simulink model "LuGre_model_BAFvsFR"  (R2026a)
settings: Solver=ode23tb  StopTime=10  MaxStep=1e-4  RelTol=1e-7  AbsTol=1e-10
model workspace (MAT data in the model file):
  omega = 40
undefined symbols (not defined in the file): Fc, Fs, k, m, sigma0, sigma1, sigma2, v_pull, vs
libraries: simulink x1
settings Model: NumberOfSteps=10  Creator=kikuchi  LastModifiedBy=kikuchi

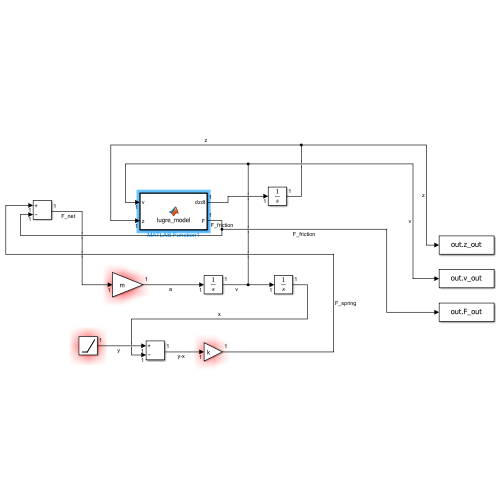
[thumbnail: Simulink's stored preview of the top-level diagram]
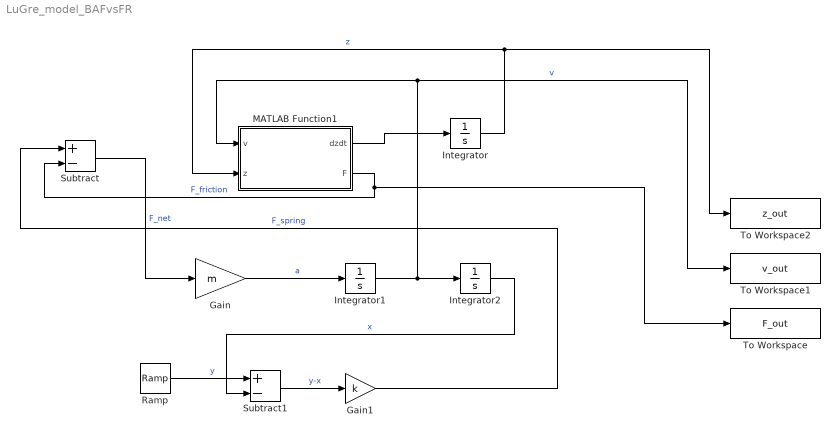
== system LuGre_model_BAFvsFR ==
  Gain : Gain  Gain=m
  Gain1 : Gain  Gain=k
  Integrator : Integrator
  Integrator1 : Integrator
  Integrator2 : Integrator
  MATLAB Function1 : MATLAB Function  TreatAsAtomicUnit=on
  Ramp : simulink/Sources/Ramp  slope=v_pull  start=0  InitialOutput=0
  Subtract : Sum  Inputs=+-
  Subtract1 : Sum  Inputs=+-
  To Workspace : ToWorkspace  VariableName=F_out  SampleTime=-1
  To Workspace1 : ToWorkspace  VariableName=v_out  SampleTime=-1
  To Workspace2 : ToWorkspace  VariableName=z_out  SampleTime=-1
  wires:
  MATLAB Function1/2(F) -> To Workspace/1, Subtract/2  "F_friction"
  Subtract/1 -> Gain/1  "F_net"
  Gain/1 -> Integrator1/1  "a"
  Integrator1/1 -> Integrator2/1, MATLAB Function1/1(v), To Workspace1/1  "v"
  Ramp/1 -> Subtract1/1  "y"
  Integrator2/1 -> Subtract1/2  "x"
  Subtract1/1 -> Gain1/1  "y-x"
  Gain1/1 -> Subtract/1  "F_spring"
  MATLAB Function1/1(dzdt) -> Integrator/1
  Integrator/1 -> MATLAB Function1/2(z), To Workspace2/1  "z"

== matlab function LuGre_model_BAFvsFR/MATLAB Function1 ==
  data: v input; dzdt output; z input; F output; sigma0 parameter; sigma1 parameter; sigma2 parameter; Fc parameter; Fs parameter; vs parameter
function [dzdt, F] = lugre_model(v, z, sigma0, sigma1, sigma2, Fc, Fs, vs)
    % parameters (from the table I in the paper of LuGre) 
    %sigma0 = 1e5; % stiffness, refined
    %sigma1 = sqrt(sigma0); % damping(減衰)
    %sigma2 = 0.4; % viscosity coefficient(粘性係数)
    %Fc = 1.0; % dynamic friction force(動摩擦力)
    %Fs = 1.5; % static friction force(静止摩擦力)
    %vs = 0.001; % stribeck speed(ストライベック速度)
    
    % g(v)
    gv = Fc + (Fs - Fc) * exp(-(v/vs)^2);
    
    % dz/dt
    dzdt = v - (sigma0 * abs(v) / gv) * z;
    
    % F
    F = sigma0 * z + sigma1 * dzdt + sigma2 * v;
end
